simulink model "model_Discrete_Kd"  (R2016b)
settings: Solver=ode45  StartTime=0.0  StopTime=12  MaxStep=1e-3  RelTol=1e-3  EnableMultiTasking=on
values from neighbouring files (symbols this model uses):
  N_bar = -inv(Cn*((A-B*K1)\B))    [pendulum.m]
undefined symbols (not defined in the file or in its folder): DiscIntNeverNeededParam, J, Kd, L, m, r
undefined symbols (not defined in the file): M
libraries: simulink x2
settings Model: Creator=Patrick  LastModifiedBy=Craig
settings DataIOCC: LimitDataPoints=on  SaveFormat=Array  SignalLoggingSaveFormat=ModelDataLogs
settings OptimizationCC: ExpressionDepthLimit=2147483647  LifeSpan=inf
settings DebuggingCC: UnderspecifiedInitializationDetection=Classic  MergeDetectMultiDrivingBlocksExec=none  SolverPrmCheckMsg=warning  FcnCallInpInsideContextMsg=warning  StateNameClashWarn=warning  SFUnexpectedBacktrackingDiag=warning  SFNoUnconditionalDefaultTransitionDiag=warning  SFExecutionAtInitializationDiag=none
settings HardwareCC: ProdBitPerPointer=32  ProdBitPerSizeT=32  ProdBitPerPtrDiffT=32  ProdLargestAtomicFloat=None  ProdIntDivRoundTo=Undefined  ProdEndianess=Unspecified  ProdWordSize=32  ProdHWDeviceType=32-bit Generic
settings ModelReferenceCC: PropagateSignalLabelsOutOfModel=off
settings GRTTargetCC: TargetLangStandard=C89/C90 (ANSI)  GeneratePreprocessorConditionals=Disable all  CombineOutputUpdateFcns=off  GRTInterface=on
settings ConfigComp: CovMetricSettings=dw  CovHtmlReporting=on  CovSaveCumulativeToWorkspaceVar=on  CovSaveSingleToWorkspaceVar=on  CovExternalEMLEnable=off

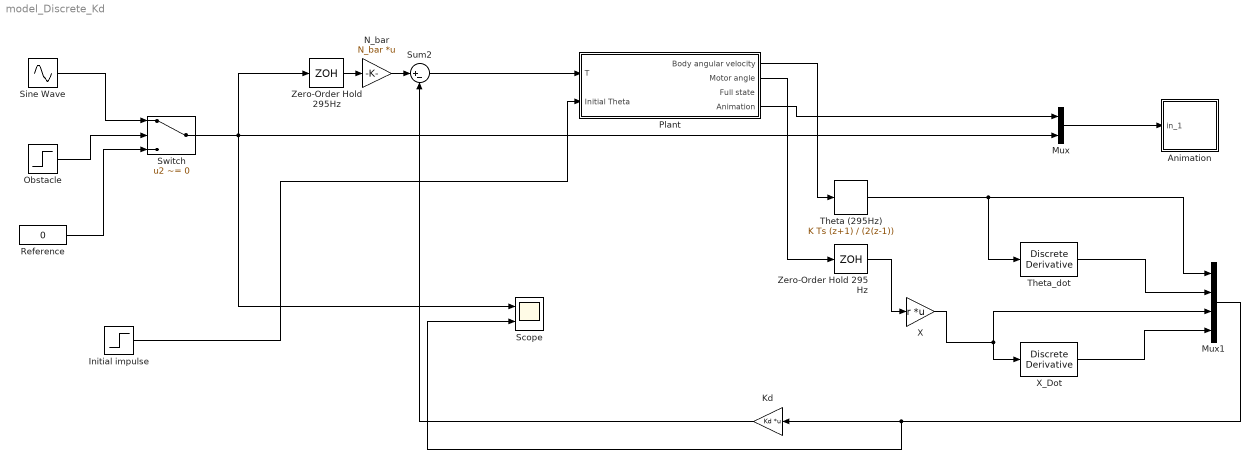
== system model_Discrete_Kd ==
  Animation : Subsystem  mask(Pendulum plot){RefBlock=Reference, L=L, r=r, Ts=1e-3}
      mask prompts: RefBlock "DC reference signal block name:"; L "Location of mass"; r "Radius of wheel"; Ts "Simulation time step"
      mask help: Pendulum plot
      mask Help: Pendulum animation function using Handle graphics.
      mask Display: plot([-10 10],[0 0],[-2 -2 2 2],[0 1 1 0],[0 3],[1 5])
  "Initial impulse " : Step  Time=5  After=0  SampleTime=0
  Kd : Gain  Gain=Kd  Multiplication=Matrix(K*u)
  Mux : Mux  Inputs=2
  Mux1 : Mux
  N_bar : Gain  Gain=N_bar  Multiplication=Matrix(K*u)
  "Obstacle " : Step  Time=2  SampleTime=0
  Plant : Subsystem  mask{m=m, mw=M, J=J, r=r, L=L, g=9.81, theta0=0.1}
      mask prompts: m "Mass of body"; mw "Mass of wheel"; J "Inertia of wheel"; r "Radius of wheel"; L "Height of body COM"; g "Gravity"; theta0 "Initial angle"
  Reference : Constant  Value=0
  Scope : Scope  NumInputPorts=2
  Sine Wave : Sin  Amplitude=0.2  Frequency=1.03  SampleTime=0
  Sum2 : Sum  Inputs=|+-
  Switch : Switch  Criteria=u2 ~= 0
  "Theta (295Hz) " : DiscreteIntegrator  IntegratorMethod=Integration: Trapezoidal  InitialConditionSetting=State (most efficient)  SampleTime=0.0034  ICPrevOutput=DiscIntNeverNeededParam  ICPrevScaledInput=DiscIntNeverNeededParam
  Theta_dot : simulink/Discrete/Discrete Derivative  gainval=1.0  ICPrevScaledInput=0.0  OutMin=[]  OutMax=[]  OutDataType=fixdt(1, 16)  OutScaling=2^-10  DoSatur=off
  X : Gain  Gain=r  Multiplication=Matrix(K*u)
  "X_Dot " : simulink/Discrete/Discrete Derivative  gainval=1.0  ICPrevScaledInput=0.0  OutMin=[]  OutMax=[]  OutDataType=fixdt(1, 16)  OutScaling=2^-10  DoSatur=off
  Zero-Order Hold 295 Hz : ZeroOrderHold  SampleTime=0.00338
  Zero-Order Hold 295Hz : ZeroOrderHold  SampleTime=0.00338
  wires:
  Plant/4(Animation) -> Mux/1
  Kd/1 -> Sum2/2
  Plant/1(Body angular velocity) -> "Theta (295Hz) "/1
  Sum2/1 -> Plant/1(T)
  Plant/2(Motor angle) -> Zero-Order Hold 295 Hz/1
  X/1 -> "X_Dot "/1, Mux1/3
  "Theta (295Hz) "/1 -> Theta_dot/1, Mux1/1
  N_bar/1 -> Sum2/1
  Mux/1 -> Animation/1(in_1)
  Theta_dot/1 -> Mux1/2
  Zero-Order Hold 295 Hz/1 -> X/1
  Zero-Order Hold 295Hz/1 -> N_bar/1
  Mux1/1 -> Scope/2, Kd/1
  "X_Dot "/1 -> Mux1/4
  "Initial impulse "/1 -> Plant/2(Initial Theta)
  Switch/1 -> Scope/1, Mux/2, Zero-Order Hold 295Hz/1
  "Obstacle "/1 -> Switch/2
  Sine Wave/1 -> Switch/1
  Reference/1 -> Switch/3

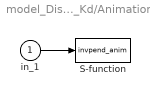
== system model_Discrete_Kd/Animation ==
  in_1 : Inport
  S-function : S-Function  FunctionName=invpend_anim  Parameters=RefBlock,L,r,Ts  SFunctionDeploymentMode=off  EnableBusSupport=off
      settings: DeleteFcn=pendan([],[],[],'DeleteBlock');
  wires:
  in_1/1 -> S-function/1

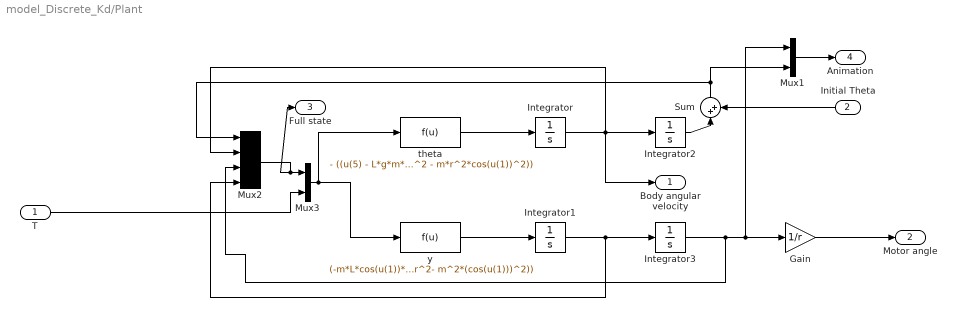
== system model_Discrete_Kd/Plant ==
  T : Inport
  Initial Theta : Inport  Port=2
  Gain : Gain  Gain=1/r
  Integrator{,1..3} (4 alike) : Integrator
  Mux1 : Mux  Inputs=2
  Mux2 : Mux
  Mux3 : Mux  Inputs=2
  Sum : Sum  Inputs=|++
  theta : Fcn  Expr=- ((u(5) - L*g*m*sin(u(1)))*(J + m*r^2 + mw*r^2))/(L^2*m*(J + m*r^2 + mw*r^2 - m*r^2*cos(u(1))^2)) - (r^2*cos(u(1))*(u(5)/r + L*m*u(2)^2*sin(u(1))))/(L*(J + m*r^2 + mw*r^2 - m*r^2*cos(u(1))^2))
  y : Fcn  Expr=(-m*L*cos(u(1))*(m*g*L*sin(u(1)) - u(5)) + m*L^2*(m*L*u(2)^2*sin(u(1))+u(5)/r))/(L^2*(m^2+m*mw+(m*J)/r^2- m^2*(cos(u(1)))^2))
  Body angular velocity : Outport
  Motor angle : Outport  Port=2
  Full state : Outport  Port=3
  Animation : Outport  Port=4
  wires:
  y/1 -> Integrator1/1
  Integrator/1 -> Body angular velocity/1, Integrator2/1, Mux2/2
  Integrator1/1 -> Integrator3/1, Mux2/4
  Integrator3/1 -> Gain/1, Mux1/1, Mux2/3
  T/1 -> Mux3/2
  Gain/1 -> Motor angle/1
  Integrator2/1 -> Sum/1
  Sum/1 -> Mux1/2, Mux2/1
  Initial Theta/1 -> Sum/2
  Mux1/1 -> Animation/1
  Mux2/1 -> Full state/1, Mux3/1
  Mux3/1 -> theta/1, y/1
  theta/1 -> Integrator/1
